simulink subsystem "MeasurementPLL"  (R2025a)
settings: Solver=VariableStepAuto  StartTime=0.0  StopTime=10.0  RelTol=1e-3
model mask{f=0, MVA=0, baseV=0}
  mask prompts: f "Grid Frequency (Hz)"; MVA "Base Power (VA)"; baseV "Base Voltage (V)"
undefined symbols (not defined in the file): Ts
libraries: eeGeneralControl x4, nesl_utility x4, ee_lib x2, eeTransforms x2, eeSinusoidalMeasurementV2 x1
settings Model: Creator=Rajarshi  LastModifiedBy=rajarshd

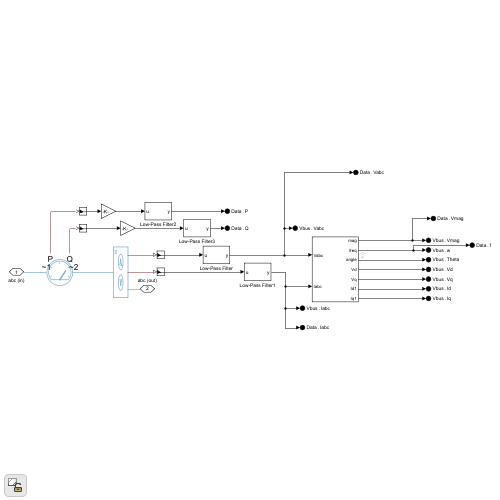
[thumbnail: Simulink's stored preview of the top-level diagram]
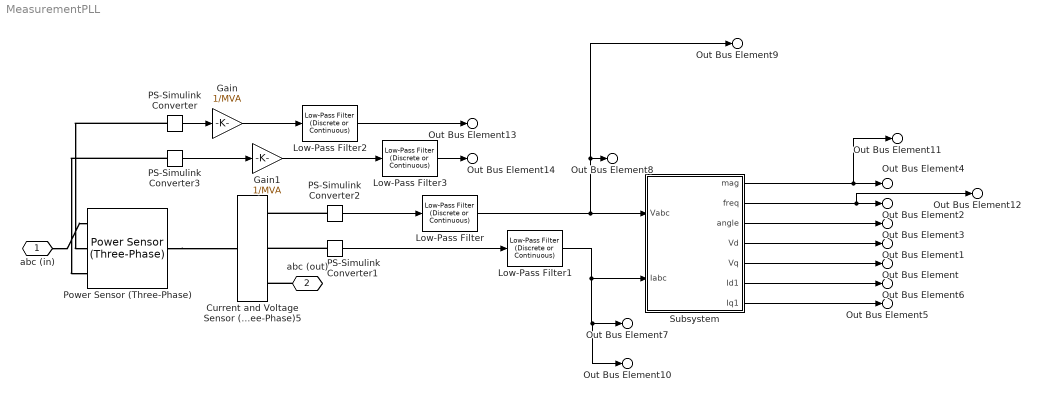
== system MeasurementPLL ==
  Current and Voltage Sensor (Three-Phase)5 : ee_lib/Sensors & Transducers/Current and Voltage Sensor (Three-Phase)  vMeasurementType=ee.enum.vmeasurement.lg  outputUnit=ee.enum.unit.pu  SRated=MVA A*V  VRated=baseV V  I_specify=off  I_priority=None  I=[0, 0, 0] A  I_nominal_specify=off  I_nominal_value=1  I_nominal_unit=A  V_specify=off  V_priority=None  V=[0, 0, 0] V  V_nominal_specify=off  V_nominal_value=1  V_nominal_unit=V
      settings: InternalSimscapePortConfiguration="{\"Bottom\":[],\"Left\":[{\"id\":\"N1\",\"label\":\"~1\",\"type\":\"foundation.electrical.three_phase\"}],\"Right\":[{\"id\":\"V_output\",\"label\":\"V\",\"type\":\"output\"},{\"id\":\"I_output\",\"label\":\"I\",\"type\":\"output\"},{\"id\":\"N2\",\"label\":\"~2\",\"type\":\"foundation.electrical.three_phase\"}],\"Top\":[]}"
  Gain : Gain  Gain=1/MVA
  Gain1 : Gain  Gain=1/MVA
  Low-Pass Filter{,1..3} (4 alike) : eeGeneralControl/Low-Pass Filter (Discrete or Continuous)  K=1  T=Ts  B=inf  A=-inf  init_option=Inherited from block input  x0=0  Ts=Ts
  PS-Simulink Converter{,1..3} (4 alike) : nesl_utility/PS-Simulink Converter  PhysicalDomain=network_engine_domain  SubClassName=ps_output  LeftPortType=input  RightPortType=output  PseudoPeriodic=off  Frequencies=[]  VectorFormat=inherit  Unit=inherit  AffineConversion=off
  Power Sensor (Three-Phase) : ee_lib/Sensors & Transducers/Power Sensor (Three-Phase)  load_type=ee.enum.passive.type_balanced.balanced  f0=60 Hz
      settings: InternalSimscapePortConfiguration="{\"Bottom\":[],\"Left\":[{\"id\":\"N1\",\"label\":\"~1\",\"type\":\"foundation.electrical.three_phase\"}],\"Right\":[{\"id\":\"N2\",\"label\":\"~2\",\"type\":\"foundation.electrical.three_phase\"}],\"Top\":[{\"id\":\"Pm\",\"label\":\"P\",\"type\":\"output\"},{\"id\":\"Qm\",\"label\":\"Q\",\"type\":\"output\"}]}"
  Subsystem : Subsystem
  abc (in) : PMIOPort  Side=Left
  abc (out) : PMIOPort  Port=2  Side=Right
  Out Bus Element : Outport  PortName=Vbus  Element=Vq
  Out Bus Element1 : Outport  PortName=Vbus  Element=Vd
  Out Bus Element2 : Outport  PortName=Vbus  Element=w
  Out Bus Element3 : Outport  PortName=Vbus  Element=Theta
  Out Bus Element4 : Outport  PortName=Vbus  Element=Vmag
  Out Bus Element5 : Outport  PortName=Vbus  Element=Iq
  Out Bus Element6 : Outport  PortName=Vbus  Element=Id
  Out Bus Element7 : Outport  PortName=Vbus  Element=Iabc
  Out Bus Element8 : Outport  PortName=Vbus  Element=Vabc
  Out Bus Element11 : Outport  Port=2  PortName=Data  Element=Vmag
  Out Bus Element12 : Outport  Port=2  PortName=Data  Element=f
  Out Bus Element10 : Outport  Port=2  PortName=Data  Element=Iabc
  Out Bus Element9 : Outport  Port=2  PortName=Data  Element=Vabc
  Out Bus Element13 : Outport  Port=2  PortName=Data  Element=P
  Out Bus Element14 : Outport  Port=2  PortName=Data  Element=Q
  wires:
  PS-Simulink Converter1/1 -> Low-Pass Filter1/1
  PS-Simulink Converter2/1 -> Low-Pass Filter/1
  Gain1/1 -> Low-Pass Filter3/1
  Low-Pass Filter/1 -> Out Bus Element9/1, Out Bus Element8/1, Subsystem/1(Vabc)
  Subsystem/1(mag) -> Out Bus Element11/1, Out Bus Element4/1
  PS-Simulink Converter3/1 -> Gain1/1
  Subsystem/4(Vd) -> Out Bus Element1/1
  Subsystem/6(Id1) -> Out Bus Element6/1
  Low-Pass Filter1/1 -> Out Bus Element10/1, Out Bus Element7/1, Subsystem/2(Iabc)
  Subsystem/3(angle) -> Out Bus Element3/1
  Gain/1 -> Low-Pass Filter2/1
  Subsystem/2(freq) -> Out Bus Element12/1, Out Bus Element2/1
  PS-Simulink Converter/1 -> Gain/1
  Low-Pass Filter3/1 -> Out Bus Element14/1
  Low-Pass Filter2/1 -> Out Bus Element13/1
  Subsystem/7(Iq1) -> Out Bus Element5/1
  Subsystem/5(Vq) -> Out Bus Element/1
  connections:
  abc (in)/RConn1 -- Power Sensor (Three-Phase)/LConn1
  Power Sensor (Three-Phase)/RConn1 -- Current and Voltage Sensor (Three-Phase)5/LConn1
  PS-Simulink Converter1/LConn1 -- Current and Voltage Sensor (Three-Phase)5/RConn2
  PS-Simulink Converter2/LConn1 -- Current and Voltage Sensor (Three-Phase)5/RConn1
  PS-Simulink Converter/LConn1 -- Power Sensor (Three-Phase)/LConn2
  abc (out)/RConn1 -- Current and Voltage Sensor (Three-Phase)5/RConn3
  PS-Simulink Converter3/LConn1 -- Power Sensor (Three-Phase)/LConn3

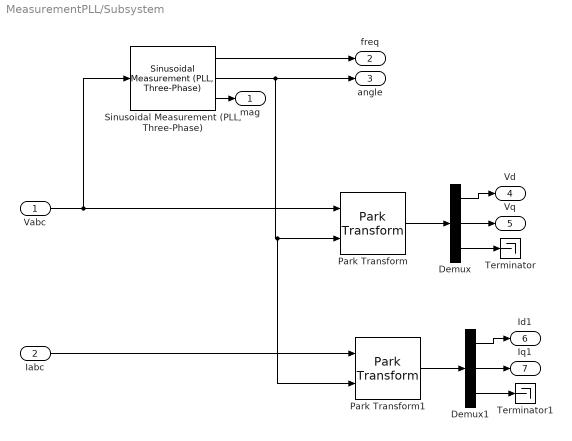
== system MeasurementPLL/Subsystem ==
  Vabc : Inport
  Iabc : Inport  Port=2
  Demux : Demux  Outputs=3
  Demux1 : Demux  Outputs=3
  Park Transform : eeTransforms/Park Transform  AxisAlignment=Q-axis  PowerInvariant=off
  Park Transform1 : eeTransforms/Park Transform  AxisAlignment=Q-axis  PowerInvariant=off
  "Sinusoidal Measurement (PLL, Three-Phase)" : eeSinusoidalMeasurementV2/Sinusoidal Measurement (PLL, Three-Phase)  InputFilter=on  InputNormalization=off  Kp_LF=100  Ki_LF=2000  F0=f  Theta0=0  Ts=-1
  Terminator : Terminator
  Terminator1 : Terminator
  mag : Outport
  freq : Outport  Port=2
  angle : Outport  Port=3
  Vd : Outport  Port=4
  Vq : Outport  Port=5
  Id1 : Outport  Port=6
  Iq1 : Outport  Port=7
  wires:
  Demux/3 -> Terminator/1
  Vabc/1 -> "Sinusoidal Measurement (PLL, Three-Phase)"/1, Park Transform/1
  Park Transform/1 -> Demux/1
  Demux/1 -> Vd/1
  Demux/2 -> Vq/1
  "Sinusoidal Measurement (PLL, Three-Phase)"/2 -> angle/1, Park Transform1/2, Park Transform/2
  "Sinusoidal Measurement (PLL, Three-Phase)"/1 -> freq/1
  "Sinusoidal Measurement (PLL, Three-Phase)"/3 -> mag/1
  Park Transform1/1 -> Demux1/1
  Demux1/1 -> Id1/1
  Demux1/2 -> Iq1/1
  Demux1/3 -> Terminator1/1
  Iabc/1 -> Park Transform1/1
